simulink library "cf_plant_lib"  (R2026a)
settings: Solver=VariableStepAuto
settings Model: Creator=user poco smart  LastModifiedBy=user poco smart

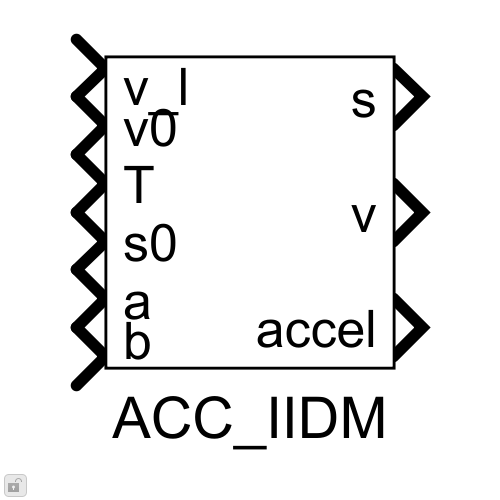
[thumbnail: Simulink's stored preview of the top-level diagram]
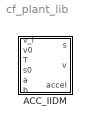
== system cf_plant_lib ==
  ACC_IIDM : Subsystem

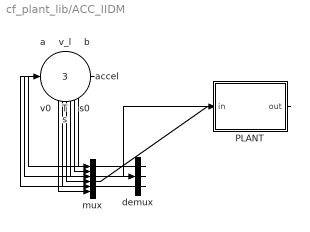
== system cf_plant_lib/ACC_IIDM ==
  v_l : Inport
  v0 : Inport  Port=2
  T : Inport  Port=3
  s0 : Inport  Port=4
  a : Inport  Port=5
  b : Inport  Port=6
  PLANT : MATLAB Function  TreatAsAtomicUnit=on
  demux : Demux  Outputs=3
  mux : Mux  Inputs=6
  s : Outport
  v : Outport  Port=2
  accel : Outport  Port=3
  wires:
  v_l/1 -> mux/1
  v0/1 -> mux/2
  T/1 -> mux/3
  s0/1 -> mux/4
  a/1 -> mux/5
  b/1 -> mux/6
  mux/1 -> PLANT/1(in)
  PLANT/1(out) -> demux/1
  demux/1 -> s/1
  demux/2 -> v/1
  demux/3 -> accel/1

== matlab function cf_plant_lib/ACC_IIDM/PLANT ==
  data: in input; out output
function out = PLANT(in)
%#codegen
% Plant ACC-IIDM self-contained. in=[v_l;v0;T;s0;a;b] (6x1), out=[s;v;accel] (3x1).
  DT = 0.1; ALPHA = exp(-DT/1.0); NORM_S_MAX = 150; COOL = 0.99;
  vl = in(1); v0 = max(in(2),1e-3); T = max(in(3),1e-3);
  s0 = in(4); a = max(in(5),1e-3); b = max(in(6),1e-3);
  persistent s v alf vlp started
  if isempty(started)
    v = 0.8*v0; s = s0 + v*T; alf = 0; vlp = vl; started = true;
  end
  % stima a_l (filtro OU su differenze finite del leader)
  alf = ALPHA*alf + (1-ALPHA)*((vl - vlp)/DT); vlp = vl;
  dv = v - vl;
  % --- acc_iidm_accel: IIDM base + CAH + blend ACC ---
  sab = max(sqrt(a*b), 1e-6);
  s_star = s0 + max(v*T + v*dv/(2*sab), 0);
  s_safe = max(s, 2.0);
  v_free = a*(1 - min(v/v0, 10)^4);
  z = min(s_star/s_safe, 20);
  below = (v <= v0);
  a_z = a*(1 - z^2);
  if z < 1
    if below, a_iidm = v_free*(1 - z^2); else, a_iidm = v_free; end
  else
    if below, a_iidm = a_z; else, a_iidm = v_free + a_z; end
  end
  a_l_bar = min(alf, a);
  a_cah = a_l_bar - max(dv,0)^2/(2*s_safe + 1e-6);
  a_cah = min(max(a_cah, -9), a);
  dd = (a_iidm - a_cah)/(b + 1e-6);
  a_blend = (1-COOL)*a_iidm + COOL*(a_cah + b*tanh(dd));
  if a_iidm >= a_cah, accel = a_iidm; else, accel = a_blend; end
  accel = min(max(accel, -9), a);
  % --- integrazione balistica (s usa la v vecchia) ---
  v_old = v;
  v = min(max(v + accel*DT, 0), 1.2*v0);
  s = min(max(s + (vl - v_old)*DT, 0.5*s0), NORM_S_MAX);
  out = [s; v; accel];
end
